simulink model "simulink"  (R2025b)
settings: Solver=VariableStepAuto  StartTime=0.0  StopTime=70.0  RelTol=1e-3
settings Model: Creator=sofic  LastModifiedBy=karla
settings DataIOCC: ReturnWorkspaceOutputs=off
settings RTWCC: GPUComputeCapability=3.5

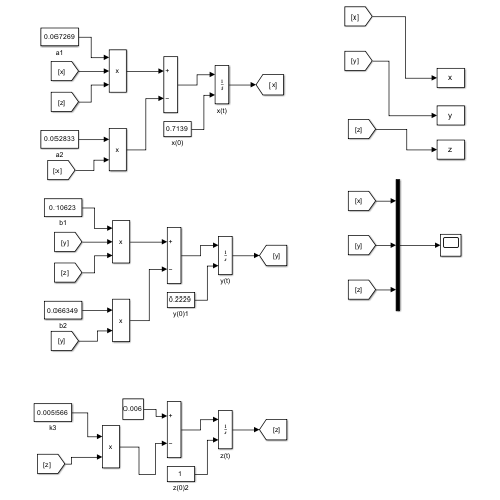
[thumbnail: Simulink's stored preview of the top-level diagram]
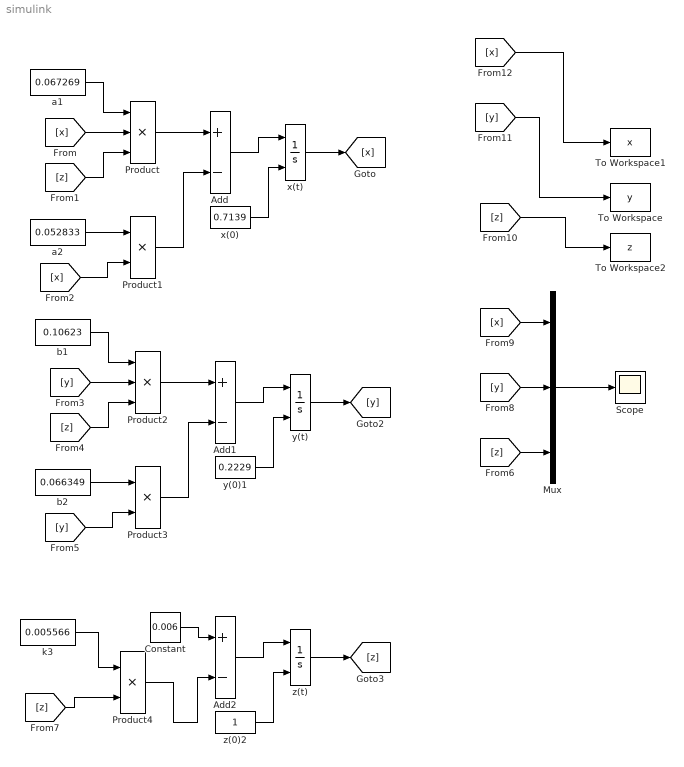
== system simulink ==
  Add : Sum  Inputs=+-
  Add1 : Sum  Inputs=+-
  Add2 : Sum  Inputs=+-
  Constant : Constant  Value=0.006
  Mux : Mux  Inputs=3
  Product : Product  Inputs=3
  Product1 : Product
  Product2 : Product  Inputs=3
  Product3 : Product
  Product4 : Product
  Scope : Scope
      settings: ActiveDisplayYMinimum=0.12410613364452408  ActiveDisplayYMaximum=1.1120447971992835
  To Workspace : ToWorkspace  VariableName=y  SampleTime=-1
  To Workspace1 : ToWorkspace  VariableName=x  SampleTime=-1
  To Workspace2 : ToWorkspace  VariableName=z  SampleTime=-1
  a1 : Constant  Value=0.067269
  a2 : Constant  Value=0.052833
  b1 : Constant  Value=0.10623
  b2 : Constant  Value=0.066349
  k3 : Constant  Value=0.005566
  x(0) : Constant  Value=0.7139
  x(t) : Integrator  InitialConditionSource=external
  y(0)1 : Constant  Value=0.2229
  y(t) : Integrator  InitialConditionSource=external
  z(0)2 : Constant
  z(t) : Integrator  InitialConditionSource=external
  wires:
  a1/1 -> Product/1
  [x] -> Product/2
  [z] -> Product/3
  Product/1 -> Add/1
  a2/1 -> Product1/1
  [x] -> Product1/2
  Product1/1 -> Add/2
  Add/1 -> x(t)/1
  x(t)/1 -> [x]
  x(0)/1 -> x(t)/2
  y(0)1/1 -> y(t)/2
  Product3/1 -> Add1/2
  b2/1 -> Product3/1
  y(t)/1 -> [y]
  Add1/1 -> y(t)/1
  Product2/1 -> Add1/1
  [y] -> Product2/2
  b1/1 -> Product2/1
  [z] -> Product2/3
  [y] -> Product3/2
  Product4/1 -> Add2/2
  z(0)2/1 -> z(t)/2
  z(t)/1 -> [z]
  Add2/1 -> z(t)/1
  k3/1 -> Product4/1
  [z] -> Product4/2
  Constant/1 -> Add2/1
  [x] -> Mux/1
  [y] -> Mux/2
  [z] -> Mux/3
  Mux/1 -> Scope/1
  [x] -> To Workspace1/1
  [y] -> To Workspace/1
  [z] -> To Workspace2/1
